simulink model "task1_motorboat_speed_control_final"  (R2024b)
settings: Solver=VariableStepAuto  StartTime=0.0  StopTime=100  RelTol=1e-3
values from neighbouring files (symbols this model uses):
  A = pi*R*R    (= 1.13097335529)    [constants_task_1.m]
  B = 0.005    [constants_task_1.m]
  D = 75    [constants_task_1.m]
  J = 0.3    [constants_task_1.m]
  k = 0.063    [constants_task_1.m]
  Kb = 0.8    [constants_task_1.m]
  Kt = 0.8    [constants_task_1.m]
  La = 0.032    [constants_task_1.m]
  M = 1200    [constants_task_1.m]
  p = 1000    [constants_task_1.m]
  Ra = 0.02    [constants_task_1.m]
libraries: slpidlib x1, simulink x1
settings Model: Creator=harih  LastModifiedBy=harih

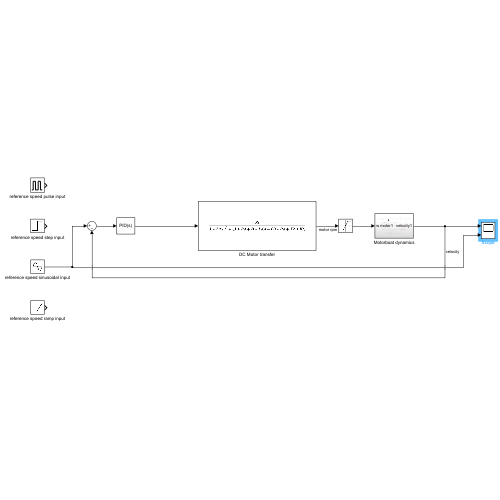
[thumbnail: Simulink's stored preview of the top-level diagram]
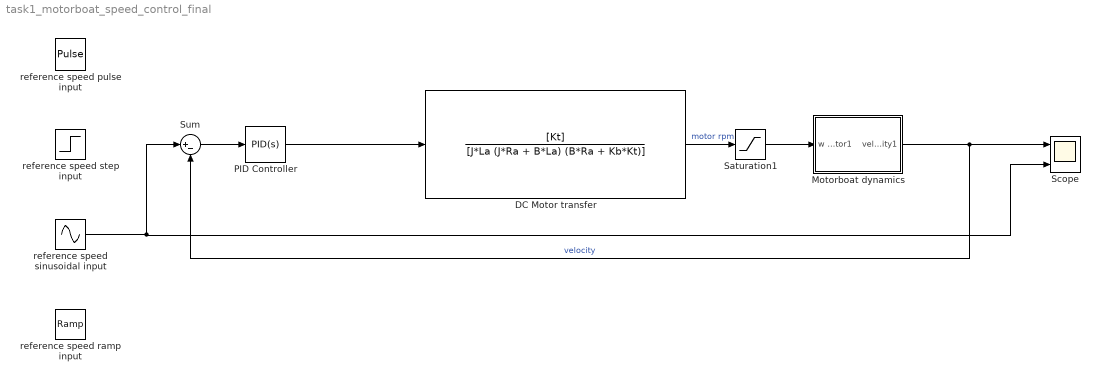
== system task1_motorboat_speed_control_final ==
  DC Motor transfer : TransferFcn  Numerator=[Kt]  Denominator=[J*La (J*Ra + B*La) (B*Ra + Kb*Kt)]
  Motorboat dynamics : Subsystem
  PID Controller : slpidlib/PID Controller  Controller=PID  Form=Parallel  TimeDomain=Continuous-time  UseExternalTs=off  SampleTime=-1  IntegratorMethod=Forward Euler  FilterMethod=Forward Euler  ControllerParametersSource=internal  P=0.0001  I=1.75  UseKiTs=off  D=0.06  UseExternalDerivativeSource=off  N=100  UseFilter=on  TunerSelectOption=Transfer Function Based (PID Tuner App)  InitialConditionSource=internal  InitialConditionForIntegrator=0  InitialConditionForFilter=0  DifferentiatorICPrevScaledInput=0  ExternalReset=none  TrackingMode=off  Kt=1  LimitOutput=off  SatLimitsSource=internal  UpperSaturationLimit=inf  LowerSaturationLimit=-inf  LinearizeAsGain=on  AntiWindupMode=none  Kb=1  LimitIntegrator=off  UpperIntegratorSaturationLimit=inf  LowerIntegratorSaturationLimit=-inf  POutMin=[]  POutMax=[]  IOutMin=[]  IOutMax=[]  DOutMin=[]  DOutMax=[]  NOutMin=[]  NOutMax=[]  SumOutMin=[]  SumOutMax=[]  SaturationOutMin=[]  SaturationOutMax=[]  PParamMin=[]  PParamMax=[]  IParamMin=[]  IParamMax=[]  DParamMin=[]  DParamMax=[]  NParamMin=[]  NParamMax=[]  KbParamMin=[]  KbParamMax=[]  KtParamMin=[]  KtParamMax=[]  KbOutMin=[]  KbOutMax=[]  KtOutMin=[]  KtOutMax=[]  IntegratorOutMin=[]  IntegratorOutMax=[]  FilterOutMin=[]  FilterOutMax=[]  SumI1OutMin=[]  SumI1OutMax=[]  SumI2OutMin=[]  SumI2OutMax=[]  SumI3OutMin=[]  SumI3OutMax=[]  SumI4OutMin=[]  SumI4OutMax=[]  SumDOutMin=[]  SumDOutMax=[]  DifferentiatorOutMin=[]  DifferentiatorOutMax=[]  FilterDiffOutCoefMin=[]  FilterDiffOutCoefMax=[]  ReciprocalOutMin=[]  ReciprocalOutMax=[]  SumDenOutMin=[]  SumDenOutMax=[]  SumNumOutMin=[]  SumNumOutMax=[]  DivideOutMin=[]  DivideOutMax=[]  UdiffTsProdOutMin=[]  UdiffTsProdOutMax=[]  NTsProdOutMin=[]  NTsProdOutMax=[]  UintegralTsProdOutMin=[]  UintegralTsProdOutMax=[]  UngainTsProdOutMin=[]  UngainTsProdOutMax=[]  ClampingZeroOutDataTypeStr=Inherit: Inherit via back propagation  ClampingZeroOutMin=[]  ClampingZeroOutMax=[]  FilterDenConstantOutDataTypeStr=Inherit: Inherit via back propagation  FilterDenConstantOutMin=[]  FilterDenConstantOutMax=[]  PCopyOutDataTypeStr=Inherit: Inherit via back propagation  PCopyOutMin=[]  PCopyOutMax=[]  NCopyOutDataTypeStr=Inherit: Inherit via back propagation  NCopyOutMin=[]  NCopyOutMax=[]  IntegratorContinuousStateAttributes=''  IntegratorStateMustResolveToSignalObject=off  IntegratorRTWStateStorageClass=Auto  FilterContinuousStateAttributes=''  FilterStateMustResolveToSignalObject=off  FilterRTWStateStorageClass=Auto  ParallelPVariant=InternalParameters  IdealPVariant=Disabled  IVariant=InternalParameters  DVariant=InternalParameters  IntegratorVariant=Continuous  SatVariant=Disabled  AWVariant=Passthrough  PCopyVariant=Disabled  TRVariant=Disabled  FdbkBlocksVariant=Forward  IdealPFdbkVariant=Disabled  SatFdbkVariant=Disabled  DerivativeFilterVariant=ContFilter  NVariant=InternalParameters  NCopyVariant=Disabled  FilterICVariant=InternalICsFilter  IntegratorICVariant=InternalICs  ExternalResetVariant=Disabled  TRSumVariant=Passthrough  SumFdbkVariant=Disabled  SumVariant=Sum_PID  TsampFilterVariant=InternalTs  TsampNgainVariant=Passthrough  TsampIntegralVariant=Disabled_SignalSpec  ExternalSaturationOutDataTypeStr=Inherit: Same as second input  DerivativeSourceVariant=ErrorSignal  PreIntVariant=InternalPreInt
  Saturation1 : Saturate  UpperLimit=314  LowerLimit=0
  Scope : Scope  NumInputPorts=2
  Sum : Sum  Inputs=|+-
  reference speed pulse input : DiscretePulseGenerator  PulseType=Time based  Period=100
  reference speed ramp input : simulink/Sources/Ramp  slope=1  start=0  InitialOutput=0
  reference speed sinusoidal input : Sin  Frequency=0.1  SampleTime=0
  reference speed step input : Step  After=100  SampleTime=0
  wires:
  reference speed sinusoidal input/1 -> Sum/1, Scope/2
  Sum/1 -> PID Controller/1
  Motorboat dynamics/1(velocity1) -> Sum/2, Scope/1  "velocity"
  PID Controller/1 -> DC Motor transfer/1
  DC Motor transfer/1 -> Saturation1/1  "motor rpm"
  Saturation1/1 -> Motorboat dynamics/1(w motor1)

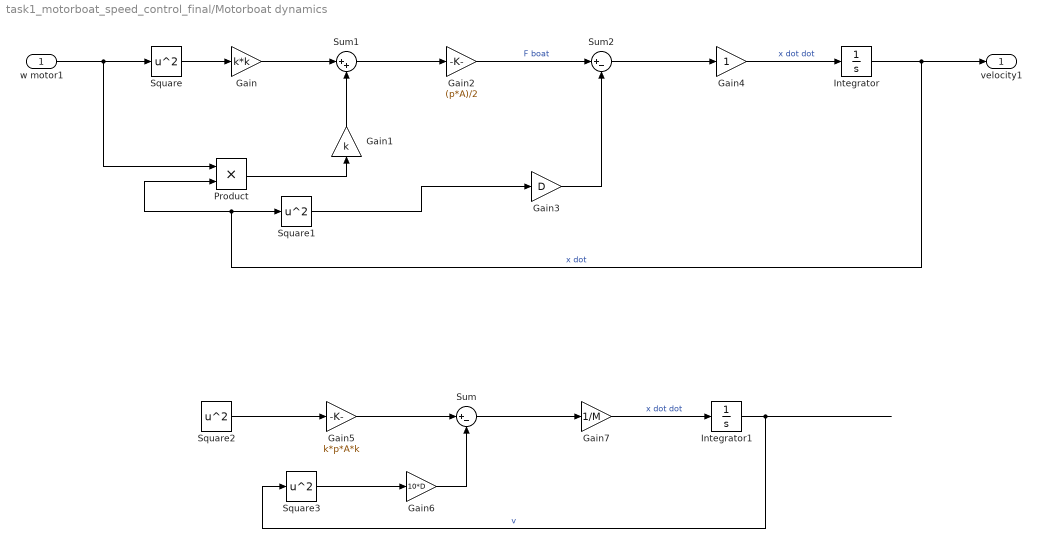
== system task1_motorboat_speed_control_final/Motorboat dynamics ==
  w motor1 : Inport
  Gain : Gain  Gain=k*k
  Gain1 : Gain  Gain=k
  Gain2 : Gain  Gain=(p*A)/2
  Gain3 : Gain  Gain=D
  Gain4 : Gain
  Gain5 : Gain  Gain=k*p*A*k
  Gain6 : Gain  Gain=10*D
  Gain7 : Gain  Gain=1/M
  Integrator : Integrator
  Integrator1 : Integrator
  Product : Product
  Square{,1..3} (4 alike) : Math  Operator=square
  Sum : Sum  Inputs=|+-
  Sum1 : Sum  Inputs=|++
  Sum2 : Sum  Inputs=|+-
  velocity1 : Outport
  wires:
  Gain3/1 -> Sum2/2
  Gain2/1 -> Sum2/1  "F boat"
  Square1/1 -> Gain3/1
  Integrator/1 -> velocity1/1, Product/2, Square1/1  "x dot"
  Gain/1 -> Sum1/1
  Square/1 -> Gain/1
  Sum2/1 -> Gain4/1
  Gain1/1 -> Sum1/2
  Gain4/1 -> Integrator/1  "x dot dot"
  Sum1/1 -> Gain2/1
  Product/1 -> Gain1/1
  ? -> Square2/1
  Square2/1 -> Gain5/1
  Gain5/1 -> Sum/1
  Gain6/1 -> Sum/2
  Square3/1 -> Gain6/1
  Sum/1 -> Gain7/1
  Gain7/1 -> Integrator1/1  "x dot dot"
  Integrator1/1 -> Square3/1  "v"
  w motor1/1 -> Product/1, Square/1
